simulink model "odw_wahadlo_z_ackerman"  (R2018b)
settings: Solver=FixedStepAuto  StartTime=0.0  StopTime=T_symulacji  FixedStep=t_krok  RelTol=1e-3
values from neighbouring files (symbols this model uses):
  b = wahadlo.b    [dane.m]    (also in dane.mat = 1)
  g = 9.80665    [dane.m]
  K = k    [opt_itae_wahadlo_ackerman.m]    (also in strojenie_wahadla_ackerman.m = K0; wahadlo_odwrocone.m = nastawy_lqr.K_lqr)
  L = wahadlo.L    [dane.m]    (also in dane.mat = 6)
  M = wahadlo.M    [dane.m]    (also in dane.mat = 5)
  m = wahadlo.m    [dane.m]    (also in dane.mat = 2)
settings Model: Creator=Admin  LastModifiedBy=Admin

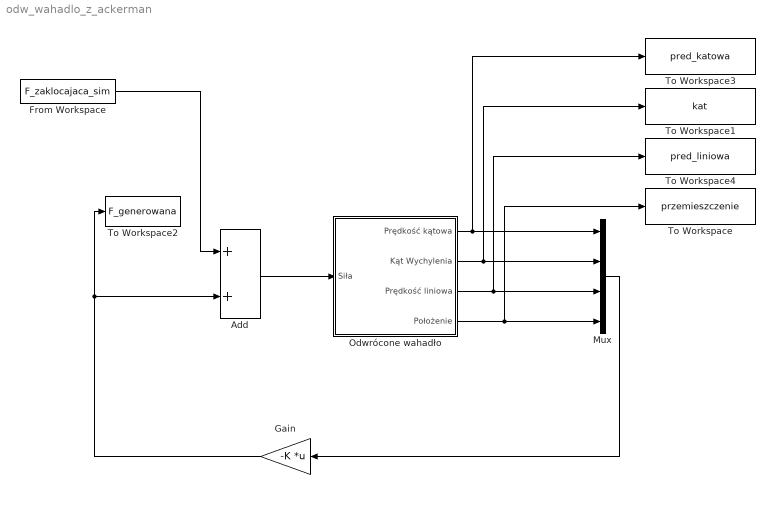
== system odw_wahadlo_z_ackerman ==
  Add : Sum
  From Workspace : FromWorkspace  VariableName=F_zaklocajaca_sim  SampleTime=0
  Gain : Gain  Gain=-K  Multiplication=Matrix(K*u)
  Mux : Mux
  "Odwrócone wahadło " : Subsystem
  To Workspace : ToWorkspace  VariableName=przemieszczenie  SampleTime=-1
  To Workspace1 : ToWorkspace  VariableName=kat  SampleTime=-1
  To Workspace2 : ToWorkspace  VariableName=F_generowana  SampleTime=-1
  To Workspace3 : ToWorkspace  VariableName=pred_katowa  SampleTime=-1
  To Workspace4 : ToWorkspace  VariableName=pred_liniowa  SampleTime=-1
  wires:
  Add/1 -> "Odwrócone wahadło "/1(Siła)
  From Workspace/1 -> Add/1
  "Odwrócone wahadło "/2(Kąt Wychylenia) -> Mux/2, To Workspace1/1
  "Odwrócone wahadło "/1(Prędkość kątowa) -> To Workspace3/1, Mux/1
  Gain/1 -> To Workspace2/1, Add/2
  Mux/1 -> Gain/1
  "Odwrócone wahadło "/3(Prędkość liniowa) -> Mux/3, To Workspace4/1
  "Odwrócone wahadło "/4(Położenie) -> Mux/4, To Workspace/1

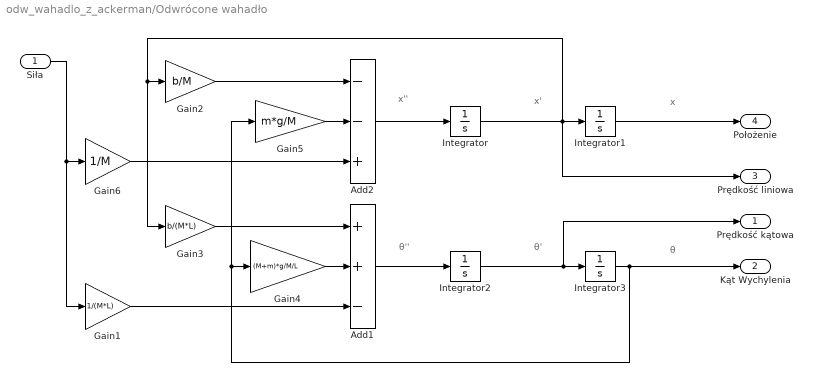
== system odw_wahadlo_z_ackerman/Odwrócone wahadło  ==
  note: θ''
  note: x''
  note: x'
  note: θ'
  note: x
  note: θ
  Siła : Inport
  Add1 : Sum  Inputs=++-
  Add2 : Sum  Inputs=--+
  Gain1 : Gain  Gain=1/(M*L)
  Gain2 : Gain  Gain=b/M
  Gain3 : Gain  Gain=b/(M*L)
  Gain4 : Gain  Gain=(M+m)*g/M/L
  Gain5 : Gain  Gain=m*g/M
  Gain6 : Gain  Gain=1/M
  Integrator{,1..3} (4 alike) : Integrator
  Prędkość kątowa : Outport
  Kąt Wychylenia : Outport  Port=2
  Prędkość liniowa : Outport  Port=3
  Położenie : Outport  Port=4
  wires:
  Integrator1/1 -> Położenie/1
  Add1/1 -> Integrator2/1
  Add2/1 -> Integrator/1
  Integrator2/1 -> Prędkość kątowa/1, Integrator3/1
  Integrator3/1 -> Kąt Wychylenia/1, Gain4/1, Gain5/1
  Gain6/1 -> Add2/3
  Siła/1 -> Gain6/1, Gain1/1
  Integrator/1 -> Prędkość liniowa/1, Integrator1/1, Gain2/1, Gain3/1
  Gain3/1 -> Add1/1
  Gain4/1 -> Add1/2
  Gain5/1 -> Add2/2
  Gain1/1 -> Add1/3
  Gain2/1 -> Add2/1
